simulink model "sim_pos_att3"  (R2018b)
settings: Solver=ode1  StartTime=0.0  StopTime=20  FixedStep=dt  RelTol=1e-3
values from neighbouring files (symbols this model uses):
  pitch = pitch - vel_forward_min_pitch    [forward_throttle_pct.m]
undefined symbols (not defined in the file or in its folder): GRAVITY_MSS, gyro_x, gyro_y, gyro_z, HD, Kd, Ku, Ld, Ldx, Ldy, Lu, Lux, Luy, m, p_angle_pitch, p_angle_yaw, pwm_max, pwm_min, Qd, Qu, roll, throttle_hover, yaw
libraries: shared6dof x1
(part 1 of 2)
settings Model: PauseTimes=0.5  Creator=a4327  LastModifiedBy=a4327
settings OptimizationCC: DefaultParameterBehavior=Inlined  UseDivisionForNetSlopeComputation=on  UseFloatMulNetSlope=on  InlineInvariantSignals=on  PassReuseOutputArgsAs=Individual arguments  ZeroExternalMemoryAtStartup=off  ZeroInternalMemoryAtStartup=off  NoFixptDivByZeroProtection=on  EfficientFloat2IntCast=on  LifeSpan=1  OptimizeBlockOrder=speed  DifferentSizesBufferReuse=on
settings DebuggingCC: ParameterTunabilityLossMsg=error
settings HardwareCC: ProdBitPerPointer=32  ProdBitPerSizeT=32  ProdBitPerPtrDiffT=32  ProdLargestAtomicFloat=None  ProdWordSize=32  ProdLongLongMode=on  ProdHWDeviceType=Custom Processor->Custom Processor
settings SFSimCC: MATLABDynamicMemAlloc=off
settings RTWCC: SystemTargetFile=ert.tlc  TemplateMakefile=ert_default_tmf  GenerateReport=on  IncludeHyperlinkInReport=on  LaunchReport=on  GenerateTraceInfo=on  GenerateTraceReport=on  GenerateTraceReportSl=on  GenerateTraceReportSf=on  GenerateTraceReportEml=on  GenerateCodeMetricsReport=on
settings CodeAppCC: ForceParamTrailComments=on  IgnoreCustomStorageClasses=off  OperatorAnnotations=on  SimulinkDataObjDesc=on  SFDataObjDesc=on  CustomSymbolStrGlobalVar=rt$N$M  CustomSymbolStrType=$N$M  CustomSymbolStrFcn=$N$M$F  CustomSymbolStrMacro=$N$M  InsertBlockDesc=on
settings ERTTargetCC: TargetLangStandard=C99 (ISO)  GenerateSampleERTMain=on  IncludeMdlTerminateFcn=off  CombineSignalStateStructs=on  SupportAbsoluteTime=off  MultiInstanceERTCode=on  CodeInterfacePackaging=Reusable function  SupportComplex=off  SupportNonInlinedSFcns=on  InlinedParameterPlacement=NonHierarchical  ERTCustomFileTemplate=example_file_process.tlc  ERTFilePackagingFormat=CompactWithDataFile

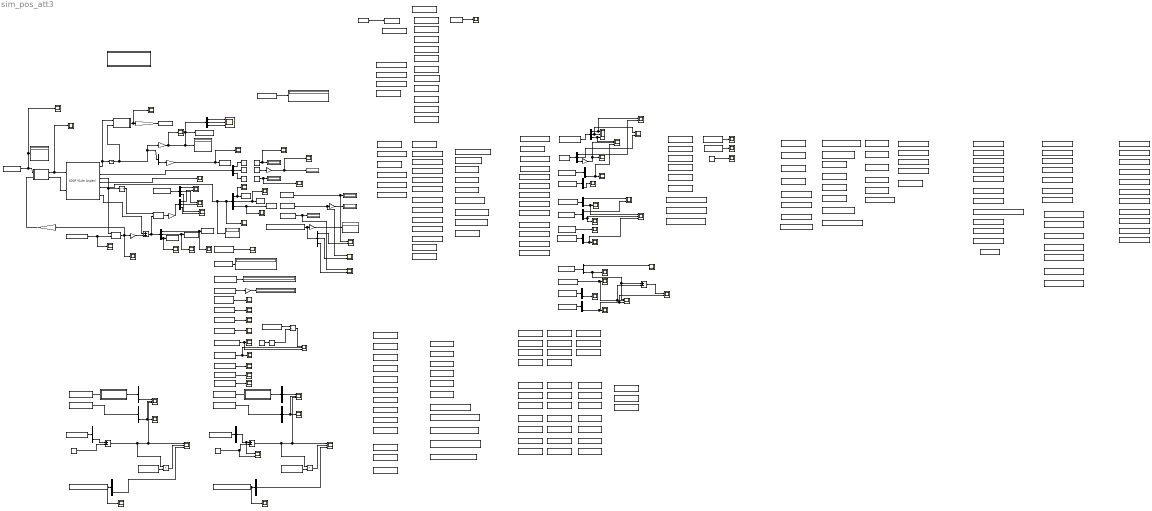
== system sim_pos_att3 ==
  6DOF (Euler Angles) : shared6dof/6DOF (Euler Angles)  units=Metric (MKS)  mtype=Fixed  rep=Euler Angles  xme_0=[0 0 0]  Vm_0=[0 0 0]  eul_0=[roll pitch yaw]  pm_0=[gyro_x gyro_y gyro_z]  mass_0=m  mass_e=0.5  mass_f=2.0  inertia=J  inertia_e=eye(3)  inertia_f=2*eye(3)  k_quat=1.0  vre_flag=on  abi_flag=off  aMode=0  xme_statename=''  Vm_statename=''  eul_statename=''  quat_statename=''  pm_statename=''  mass_statename=''
      settings: SourceProductBaseCode=AE
  AC_ATTITUDE_ACCEL_RP_CONTROLLER_MAX_RADSS : DataStoreMemory  DataStoreName=AC_ATTITUDE_ACCEL_RP_CONTROLLER_MAX_RADSS  ReadBeforeWriteMsg=warning  WriteAfterWriteMsg=warning  WriteAfterReadMsg=warning  InitialValue=AC_ATTITUDE_ACCEL_RP_CONTROLLER_MAX_RADSS  VectorParams1D=off  ShowAdditionalParam=off  OutDataTypeStr=double
  AC_ATTITUDE_ACCEL_RP_CONTROLLER_MIN_RADSS : DataStoreMemory  DataStoreName=AC_ATTITUDE_ACCEL_RP_CONTROLLER_MIN_RADSS  ReadBeforeWriteMsg=warning  WriteAfterWriteMsg=warning  WriteAfterReadMsg=warning  InitialValue=AC_ATTITUDE_ACCEL_RP_CONTROLLER_MIN_RADSS  VectorParams1D=off  ShowAdditionalParam=off  OutDataTypeStr=double
  AC_ATTITUDE_ACCEL_Y_CONTROLLER_MAX_RADSS : DataStoreMemory  DataStoreName=AC_ATTITUDE_ACCEL_Y_CONTROLLER_MAX_RADSS  ReadBeforeWriteMsg=warning  WriteAfterWriteMsg=warning  WriteAfterReadMsg=warning  InitialValue=AC_ATTITUDE_ACCEL_Y_CONTROLLER_MAX_RADSS  ShowAdditionalParam=off  OutDataTypeStr=double
  AC_ATTITUDE_ACCEL_Y_CONTROLLER_MIN_RADSS : DataStoreMemory  DataStoreName=AC_ATTITUDE_ACCEL_Y_CONTROLLER_MIN_RADSS  ReadBeforeWriteMsg=warning  WriteAfterWriteMsg=warning  WriteAfterReadMsg=warning  InitialValue=AC_ATTITUDE_ACCEL_Y_CONTROLLER_MIN_RADSS  VectorParams1D=off  ShowAdditionalParam=off  OutDataTypeStr=double
  AC_ATTITUDE_CONTROL_ANGLE_LIMIT_THROTTLE_MAX : DataStoreMemory  DataStoreName=AC_ATTITUDE_CONTROL_ANGLE_LIMIT_THROTTLE_MAX  ReadBeforeWriteMsg=warning  WriteAfterWriteMsg=warning  WriteAfterReadMsg=warning  InitialValue=AC_ATTITUDE_CONTROL_ANGLE_LIMIT_THROTTLE_MAX  VectorParams1D=off  ShowAdditionalParam=off  OutDataTypeStr=double
  AC_ATTITUDE_CONTROL_MAX : DataStoreMemory  DataStoreName=AC_ATTITUDE_CONTROL_MAX  ReadBeforeWriteMsg=warning  WriteAfterWriteMsg=warning  WriteAfterReadMsg=warning  InitialValue=AC_ATTITUDE_CONTROL_MAX  VectorParams1D=off  ShowAdditionalParam=off  OutDataTypeStr=double
  AC_ATTITUDE_THRUST_ERROR_ANGLE : DataStoreMemory  DataStoreName=AC_ATTITUDE_THRUST_ERROR_ANGLE  ReadBeforeWriteMsg=warning  WriteAfterWriteMsg=warning  WriteAfterReadMsg=warning  InitialValue=AC_ATTITUDE_THRUST_ERROR_ANGLE  ShowAdditionalParam=off  OutDataTypeStr=double
  AP_MOTORS_MATRIX_YAW_FACTOR_CCW : DataStoreMemory  DataStoreName=AP_MOTORS_MATRIX_YAW_FACTOR_CCW  ReadBeforeWriteMsg=warning  WriteAfterWriteMsg=warning  WriteAfterReadMsg=warning  InitialValue=AP_MOTORS_MATRIX_YAW_FACTOR_CCW  VectorParams1D=off  ShowAdditionalParam=off  OutDataTypeStr=double
  AP_MOTORS_MATRIX_YAW_FACTOR_CW : DataStoreMemory  DataStoreName=AP_MOTORS_MATRIX_YAW_FACTOR_CW  ReadBeforeWriteMsg=warning  WriteAfterWriteMsg=warning  WriteAfterReadMsg=warning  InitialValue=AP_MOTORS_MATRIX_YAW_FACTOR_CW  VectorParams1D=off  ShowAdditionalParam=off  OutDataTypeStr=double
  ATC_RAT_PIT_D : DataStoreMemory  DataStoreName=ATC_RAT_PIT_D  ReadBeforeWriteMsg=warning  WriteAfterWriteMsg=warning  WriteAfterReadMsg=warning  InitialValue=ATC_RAT_PIT_D  VectorParams1D=off  ShowAdditionalParam=off  OutDataTypeStr=double
  ATC_RAT_PIT_FF : DataStoreMemory  DataStoreName=ATC_RAT_PIT_FF  ReadBeforeWriteMsg=warning  WriteAfterWriteMsg=warning  WriteAfterReadMsg=warning  InitialValue=ATC_RAT_PIT_FF  VectorParams1D=off  ShowAdditionalParam=off  OutDataTypeStr=double
  ATC_RAT_PIT_FILT : DataStoreMemory  DataStoreName=ATC_RAT_PIT_FILT  ReadBeforeWriteMsg=warning  WriteAfterWriteMsg=warning  WriteAfterReadMsg=warning  InitialValue=ATC_RAT_PIT_FILT  VectorParams1D=off  ShowAdditionalParam=off  OutDataTypeStr=double
  ATC_RAT_PIT_I : DataStoreMemory  DataStoreName=ATC_RAT_PIT_I  ReadBeforeWriteMsg=warning  WriteAfterWriteMsg=warning  WriteAfterReadMsg=warning  InitialValue=ATC_RAT_PIT_I  VectorParams1D=off  ShowAdditionalParam=off  OutDataTypeStr=double
  ATC_RAT_PIT_IMAX : DataStoreMemory  DataStoreName=ATC_RAT_PIT_IMAX  ReadBeforeWriteMsg=warning  WriteAfterWriteMsg=warning  WriteAfterReadMsg=warning  InitialValue=ATC_RAT_PIT_IMAX  VectorParams1D=off  ShowAdditionalParam=off  OutDataTypeStr=double
  ATC_RAT_PIT_P : DataStoreMemory  DataStoreName=ATC_RAT_PIT_P  ReadBeforeWriteMsg=warning  WriteAfterWriteMsg=warning  WriteAfterReadMsg=warning  InitialValue=ATC_RAT_PIT_P  VectorParams1D=off  ShowAdditionalParam=off  OutDataTypeStr=double
  ATC_RAT_RLL_D : DataStoreMemory  DataStoreName=ATC_RAT_RLL_D  ReadBeforeWriteMsg=warning  WriteAfterWriteMsg=warning  WriteAfterReadMsg=warning  InitialValue=ATC_RAT_RLL_D  VectorParams1D=off  ShowAdditionalParam=off  OutDataTypeStr=double
  ATC_RAT_RLL_FF : DataStoreMemory  DataStoreName=ATC_RAT_RLL_FF  ReadBeforeWriteMsg=warning  WriteAfterWriteMsg=warning  WriteAfterReadMsg=warning  InitialValue=ATC_RAT_RLL_FF  VectorParams1D=off  ShowAdditionalParam=off  OutDataTypeStr=double
  ATC_RAT_RLL_FILT : DataStoreMemory  DataStoreName=ATC_RAT_RLL_FILT  ReadBeforeWriteMsg=warning  WriteAfterWriteMsg=warning  WriteAfterReadMsg=warning  InitialValue=ATC_RAT_RLL_FILT  VectorParams1D=off  ShowAdditionalParam=off  OutDataTypeStr=double
  ATC_RAT_RLL_I : DataStoreMemory  DataStoreName=ATC_RAT_RLL_I  ReadBeforeWriteMsg=warning  WriteAfterWriteMsg=warning  WriteAfterReadMsg=warning  InitialValue=ATC_RAT_RLL_I  VectorParams1D=off  ShowAdditionalParam=off  OutDataTypeStr=double
  ATC_RAT_RLL_IMAX : DataStoreMemory  DataStoreName=ATC_RAT_RLL_IMAX  ReadBeforeWriteMsg=warning  WriteAfterWriteMsg=warning  WriteAfterReadMsg=warning  InitialValue=ATC_RAT_RLL_IMAX  VectorParams1D=off  ShowAdditionalParam=off  OutDataTypeStr=double
  ATC_RAT_RLL_P : DataStoreMemory  DataStoreName=ATC_RAT_RLL_P  ReadBeforeWriteMsg=warning  WriteAfterWriteMsg=warning  WriteAfterReadMsg=warning  InitialValue=ATC_RAT_RLL_P  VectorParams1D=off  ShowAdditionalParam=off  OutDataTypeStr=double
  ATC_RAT_YAW_D : DataStoreMemory  DataStoreName=ATC_RAT_YAW_D  ReadBeforeWriteMsg=warning  WriteAfterWriteMsg=warning  WriteAfterReadMsg=warning  InitialValue=ATC_RAT_YAW_D  VectorParams1D=off  ShowAdditionalParam=off  OutDataTypeStr=double
  ATC_RAT_YAW_FF : DataStoreMemory  DataStoreName=ATC_RAT_YAW_FF  ReadBeforeWriteMsg=warning  WriteAfterWriteMsg=warning  WriteAfterReadMsg=warning  InitialValue=ATC_RAT_YAW_FF  VectorParams1D=off  ShowAdditionalParam=off  OutDataTypeStr=double
  ATC_RAT_YAW_FILT : DataStoreMemory  DataStoreName=ATC_RAT_YAW_FILT  ReadBeforeWriteMsg=warning  WriteAfterWriteMsg=warning  WriteAfterReadMsg=warning  InitialValue=ATC_RAT_YAW_FILT  VectorParams1D=off  ShowAdditionalParam=off  OutDataTypeStr=double
  ATC_RAT_YAW_I : DataStoreMemory  DataStoreName=ATC_RAT_YAW_I  ReadBeforeWriteMsg=warning  WriteAfterWriteMsg=warning  WriteAfterReadMsg=warning  InitialValue=ATC_RAT_YAW_I  VectorParams1D=off  ShowAdditionalParam=off  OutDataTypeStr=double
  ATC_RAT_YAW_IMAX : DataStoreMemory  DataStoreName=ATC_RAT_YAW_IMAX  ReadBeforeWriteMsg=warning  WriteAfterWriteMsg=warning  WriteAfterReadMsg=warning  InitialValue=ATC_RAT_YAW_IMAX  VectorParams1D=off  ShowAdditionalParam=off  OutDataTypeStr=double
  ATC_RAT_YAW_P : DataStoreMemory  DataStoreName=ATC_RAT_YAW_P  ReadBeforeWriteMsg=warning  WriteAfterWriteMsg=warning  WriteAfterReadMsg=warning  InitialValue=ATC_RAT_YAW_P  VectorParams1D=off  ShowAdditionalParam=off  OutDataTypeStr=double
  Add : Sum  Inputs=+-
  Add1 : Sum  Inputs=+-
  Add2 : Sum  Inputs=+-
  Add3 : Sum
  Constant : Constant  Value=p_angle_pitch
  Constant1 : Constant  Value=p_angle_yaw
  Constant2 : Constant  Value=throttle_hover
  Constant3 : Constant  Value=0.4816
  Cos : Trigonometry  Operator=cos
  Data Store Read : DataStoreRead  DataStoreName=pwm_out
  Data Store Read1 : DataStoreRead  DataStoreName=pitch
  Data Store Read10 : DataStoreRead  DataStoreName=gyro_y
  Data Store Read11 : DataStoreRead  DataStoreName=gyro_z
  Data Store Read{9,12,26,31} (4 alike) : DataStoreRead  DataStoreName=rate_target_ang_vel
  Data Store Read13 : DataStoreRead  DataStoreName=pitch_in
  Data Store Read14 : DataStoreRead  DataStoreName=roll_in
  Data Store Read15 : DataStoreRead  DataStoreName=yaw_in
  Data Store Read16 : DataStoreRead  DataStoreName=throttle_filter
  Data Store Read17 : DataStoreRead  DataStoreName=thrust_rpyt_out
  Data Store Read{7,18,25,30} (4 alike) : DataStoreRead  DataStoreName=attitude_target_euler_angle
  Data Store Read19 : DataStoreRead  DataStoreName=throttle_in
  Data Store Read2 : DataStoreRead  DataStoreName=roll
  Data Store Read20 : DataStoreRead  DataStoreName=attitude_target_euler_rate
  Data Store Read21 : DataStoreRead  DataStoreName=attitude_target_ang_vel
  Data Store Read22 : DataStoreRead  DataStoreName=attitude_ang_error
  Data Store Read23 : DataStoreRead  DataStoreName=attitude_error_vector
  Data Store Read24 : DataStoreRead  DataStoreName=pitch
  Data Store Read27 : DataStoreRead  DataStoreName=attitude_ang_error
  Data Store Read28 : DataStoreRead  DataStoreName=attitude_error_vector
  Data Store Read29 : DataStoreRead  DataStoreName=yaw
  Data Store Read3 : DataStoreRead  DataStoreName=yaw
  Data Store Read32 : DataStoreRead  DataStoreName=leash_up_z
  Data Store Read33 : DataStoreRead  DataStoreName=leash_down_z
  Data Store Read34 : DataStoreRead  DataStoreName=pos_target
  Data Store Read35 : DataStoreRead  DataStoreName=accel_target
  Data Store Read36 : DataStoreRead  DataStoreName=pos_error
  Data Store Read37 : DataStoreRead  DataStoreName=vel_target
  Data Store Read38 : DataStoreRead  DataStoreName=curr_vel
  Data Store Read39 : DataStoreRead  DataStoreName=vel_desired
  Data Store Read4 : DataStoreRead  DataStoreName=rot_body_to_ned
  Data Store Read40 : DataStoreRead  DataStoreName=vel_last
  Data Store Read41 : DataStoreRead  DataStoreName=vel_error
  Data Store Read42 : DataStoreRead  DataStoreName=accel_target
  Data Store Read43 : DataStoreRead  DataStoreName=z_accel_meas
  Data Store Read44 : DataStoreRead  DataStoreName=accel_desired
  Data Store Read45 : DataStoreRead  DataStoreName=accel_error
  Data Store Read46 : DataStoreRead  DataStoreName=leash
  Data Store Read47 : DataStoreRead  DataStoreName=angle_boost
  Data Store Read48 : DataStoreRead  DataStoreName=pitch
  Data Store Read49 : DataStoreRead  DataStoreName=throttle_in
  Data Store Read5 : DataStoreRead  DataStoreName=rot_body_to_ned
  Data Store Read50 : DataStoreRead  DataStoreName=curr_pos
  Data Store Read6 : DataStoreRead  DataStoreName=attitude_target_quat
  Data Store Read8 : DataStoreRead  DataStoreName=gyro_x
  Data Store Write : DataStoreWrite  DataStoreName=throttle_in
  Data Store Write1 : DataStoreWrite  DataStoreName=roll
  Data Store Write10 : DataStoreWrite  DataStoreName=curr_pos
  Data Store Write11 : DataStoreWrite  DataStoreName=accel_y
  Data Store Write12 : DataStoreWrite  DataStoreName=accel_x
  Data Store Write2 : DataStoreWrite  DataStoreName=yaw
  Data Store Write3 : DataStoreWrite  DataStoreName=pitch
  Data Store Write4 : DataStoreWrite  DataStoreName=gyro_x
  Data Store Write5 : DataStoreWrite  DataStoreName=gyro_y
  Data Store Write6 : DataStoreWrite  DataStoreName=gyro_z
  Data Store Write7 : DataStoreWrite  DataStoreName=curr_alt
  Data Store Write8 : DataStoreWrite  DataStoreName=accel_z
  Data Store Write9 : DataStoreWrite  DataStoreName=curr_vel
  Demux{,1..25} (26 alike) : Demux  Outputs=3
  Display{1..2,4..5,7,10..18} (14 alike) : Display
      Display7 settings: Format=bank
  Divide : Product  Inputs=*/
  GRAVITY_MSS : DataStoreMemory  DataStoreName=GRAVITY_MSS  ReadBeforeWriteMsg=warning  WriteAfterWriteMsg=warning  WriteAfterReadMsg=warning  InitialValue=GRAVITY_MSS  VectorParams1D=off  ShowAdditionalParam=off  OutDataTypeStr=double
  Gain{,1..3} (4 alike) : Gain  Gain=HD
  Gain4 : Gain  Gain=-100
  Gain5 : Gain  Gain=[100 100 -100]
  Gain6 : Gain  Gain=-1
  Gain7 : Gain  Gain=100
  Gain8 : Gain  Gain=-1
  Gain9 : Gain  Gain=100
  Gravity in Earth Axes : Gain  Gain=m  SaturateOnIntegerOverflow=on  OutDataTypeStr=Inherit: Same as input  ParamDataTypeStr=Inherit: Same as input
  Inertial to Body : Product  Multiplication=Matrix(*)  SaturateOnIntegerOverflow=on  InputSameDT=on  OutDataTypeStr=Inherit: Same as first input
  Inertial to NED : Product  Multiplication=Matrix(*)  SaturateOnIntegerOverflow=on  InputSameDT=on  OutDataTypeStr=Inherit: Same as first input
  Kx : DataStoreMemory  DataStoreName=Kx  ReadBeforeWriteMsg=warning  WriteAfterWriteMsg=warning  WriteAfterReadMsg=warning  InitialValue=Kx  VectorParams1D=off  ShowAdditionalParam=off  OutDataTypeStr=double
  MATLAB Function : MATLAB Function  TreatAsAtomicUnit=on
  MATLAB Function1 : MATLAB Function  TreatAsAtomicUnit=on
  MATLAB Function2 : MATLAB Function  TreatAsAtomicUnit=on
  POSCONTROL_ACCELERATION_MIN : DataStoreMemory  DataStoreName=POSCONTROL_ACCELERATION_MIN  ReadBeforeWriteMsg=warning  WriteAfterWriteMsg=warning  WriteAfterReadMsg=warning  InitialValue=POSCONTROL_ACCELERATION_MIN  ShowAdditionalParam=off  OutDataTypeStr=double
  POSCONTROL_ACCEL_FILTER_HZ : DataStoreMemory  DataStoreName=POSCONTROL_ACCEL_FILTER_HZ  ReadBeforeWriteMsg=warning  WriteAfterWriteMsg=warning  WriteAfterReadMsg=warning  InitialValue=POSCONTROL_ACCEL_FILTER_HZ  VectorParams1D=off  ShowAdditionalParam=off  OutDataTypeStr=double
  POSCONTROL_ACCEL_XY : DataStoreMemory  DataStoreName=POSCONTROL_ACCEL_XY  ReadBeforeWriteMsg=warning  WriteAfterWriteMsg=warning  WriteAfterReadMsg=warning  InitialValue=POSCONTROL_ACCEL_XY  VectorParams1D=off  ShowAdditionalParam=off  OutDataTypeStr=double
  POSCONTROL_ACCEL_XY_MAX : DataStoreMemory  DataStoreName=POSCONTROL_ACCEL_XY_MAX  ReadBeforeWriteMsg=warning  WriteAfterWriteMsg=warning  WriteAfterReadMsg=warning  InitialValue=POSCONTROL_ACCEL_XY_MAX  VectorParams1D=off  ShowAdditionalParam=off  OutDataTypeStr=double
  POSCONTROL_ACCEL_Z : DataStoreMemory  DataStoreName=POSCONTROL_ACCEL_Z  ReadBeforeWriteMsg=warning  WriteAfterWriteMsg=warning  WriteAfterReadMsg=warning  InitialValue=POSCONTROL_ACCEL_Z  ShowAdditionalParam=off  OutDataTypeStr=double
  POSCONTROL_ACC_Z_D : DataStoreMemory  DataStoreName=POSCONTROL_ACC_Z_D  ReadBeforeWriteMsg=warning  WriteAfterWriteMsg=warning  WriteAfterReadMsg=warning  InitialValue=POSCONTROL_ACC_Z_D  VectorParams1D=off  ShowAdditionalParam=off  OutDataTypeStr=double
  POSCONTROL_ACC_Z_FILT_HZ : DataStoreMemory  DataStoreName=POSCONTROL_ACC_Z_FILT_HZ  ReadBeforeWriteMsg=warning  WriteAfterWriteMsg=warning  WriteAfterReadMsg=warning  InitialValue=POSCONTROL_ACC_Z_FILT_HZ  VectorParams1D=off  ShowAdditionalParam=off  OutDataTypeStr=double
  POSCONTROL_ACC_Z_I : DataStoreMemory  DataStoreName=POSCONTROL_ACC_Z_I  ReadBeforeWriteMsg=warning  WriteAfterWriteMsg=warning  WriteAfterReadMsg=warning  InitialValue=POSCONTROL_ACC_Z_I  VectorParams1D=off  ShowAdditionalParam=off  OutDataTypeStr=double
  POSCONTROL_ACC_Z_IMAX : DataStoreMemory  DataStoreName=POSCONTROL_ACC_Z_IMAX  ReadBeforeWriteMsg=warning  WriteAfterWriteMsg=warning  WriteAfterReadMsg=warning  InitialValue=POSCONTROL_ACC_Z_IMAX  VectorParams1D=off  ShowAdditionalParam=off  OutDataTypeStr=double
  POSCONTROL_ACC_Z_P : DataStoreMemory  DataStoreName=POSCONTROL_ACC_Z_P  ReadBeforeWriteMsg=warning  WriteAfterWriteMsg=warning  WriteAfterReadMsg=warning  InitialValue=POSCONTROL_ACC_Z_P  VectorParams1D=off  ShowAdditionalParam=off  OutDataTypeStr=double
  POSCONTROL_JERK_RATIO : DataStoreMemory  DataStoreName=POSCONTROL_JERK_RATIO  ReadBeforeWriteMsg=warning  WriteAfterWriteMsg=warning  WriteAfterReadMsg=warning  InitialValue=POSCONTROL_JERK_RATIO  VectorParams1D=off  ShowAdditionalParam=off  OutDataTypeStr=double
  POSCONTROL_LEASH_LENGTH_MIN : DataStoreMemory  DataStoreName=POSCONTROL_LEASH_LENGTH_MIN  ReadBeforeWriteMsg=warning  WriteAfterWriteMsg=warning  WriteAfterReadMsg=warning  InitialValue=POSCONTROL_LEASH_LENGTH_MIN  VectorParams1D=off  ShowAdditionalParam=off  OutDataTypeStr=double
  POSCONTROL_OVERSPEED_GAIN_Z : DataStoreMemory  DataStoreName=POSCONTROL_OVERSPEED_GAIN_Z  ReadBeforeWriteMsg=warning  WriteAfterWriteMsg=warning  WriteAfterReadMsg=warning  InitialValue=POSCONTROL_OVERSPEED_GAIN_Z  VectorParams1D=off  ShowAdditionalParam=off  OutDataTypeStr=double
  POSCONTROL_POS_XY_P : DataStoreMemory  DataStoreName=POSCONTROL_POS_XY_P  ReadBeforeWriteMsg=warning  WriteAfterWriteMsg=warning  WriteAfterReadMsg=warning  InitialValue=POSCONTROL_POS_XY_P  VectorParams1D=off  ShowAdditionalParam=off  OutDataTypeStr=double
  POSCONTROL_POS_Z_P : DataStoreMemory  DataStoreName=POSCONTROL_POS_Z_P  ReadBeforeWriteMsg=warning  WriteAfterWriteMsg=warning  WriteAfterReadMsg=warning  InitialValue=POSCONTROL_POS_Z_P  VectorParams1D=off  ShowAdditionalParam=off  OutDataTypeStr=double
  POSCONTROL_SPEED : DataStoreMemory  DataStoreName=POSCONTROL_SPEED  ReadBeforeWriteMsg=warning  WriteAfterWriteMsg=warning  WriteAfterReadMsg=warning  InitialValue=POSCONTROL_SPEED  ShowAdditionalParam=off  OutDataTypeStr=double
  POSCONTROL_SPEED_DOWN : DataStoreMemory  DataStoreName=POSCONTROL_SPEED_DOWN  ReadBeforeWriteMsg=warning  WriteAfterWriteMsg=warning  WriteAfterReadMsg=warning  InitialValue=POSCONTROL_SPEED_DOWN  ShowAdditionalParam=off  OutDataTypeStr=double
  POSCONTROL_SPEED_UP : DataStoreMemory  DataStoreName=POSCONTROL_SPEED_UP  ReadBeforeWriteMsg=warning  WriteAfterWriteMsg=warning  WriteAfterReadMsg=warning  InitialValue=POSCONTROL_SPEED_UP  ShowAdditionalParam=off  OutDataTypeStr=double
  POSCONTROL_STOPPING_DIST_DOWN_MAX : DataStoreMemory  DataStoreName=POSCONTROL_STOPPING_DIST_DOWN_MAX  ReadBeforeWriteMsg=warning  WriteAfterWriteMsg=warning  WriteAfterReadMsg=warning  InitialValue=POSCONTROL_STOPPING_DIST_DOWN_MAX  VectorParams1D=off  ShowAdditionalParam=off  OutDataTypeStr=double
  POSCONTROL_STOPPING_DIST_UP_MAX : DataStoreMemory  DataStoreName=POSCONTROL_STOPPING_DIST_UP_MAX  ReadBeforeWriteMsg=warning  WriteAfterWriteMsg=warning  WriteAfterReadMsg=warning  InitialValue=POSCONTROL_STOPPING_DIST_UP_MAX  VectorParams1D=off  ShowAdditionalParam=off  OutDataTypeStr=double
  POSCONTROL_THROTTLE_CUTOFF_FREQ : DataStoreMemory  DataStoreName=POSCONTROL_THROTTLE_CUTOFF_FREQ  ReadBeforeWriteMsg=warning  WriteAfterWriteMsg=warning  WriteAfterReadMsg=warning  InitialValue=POSCONTROL_THROTTLE_CUTOFF_FREQ  VectorParams1D=off  ShowAdditionalParam=off  OutDataTypeStr=double
  POSCONTROL_VEL_ERROR_CUTOFF_FREQ : DataStoreMemory  DataStoreName=POSCONTROL_VEL_ERROR_CUTOFF_FREQ  ReadBeforeWriteMsg=warning  WriteAfterWriteMsg=warning  WriteAfterReadMsg=warning  InitialValue=POSCONTROL_VEL_ERROR_CUTOFF_FREQ  VectorParams1D=off  ShowAdditionalParam=off  OutDataTypeStr=double
  POSCONTROL_VEL_XY_D : DataStoreMemory  DataStoreName=POSCONTROL_VEL_XY_D  ReadBeforeWriteMsg=warning  WriteAfterWriteMsg=warning  WriteAfterReadMsg=warning  InitialValue=POSCONTROL_VEL_XY_D  VectorParams1D=off  ShowAdditionalParam=off  OutDataTypeStr=double
  POSCONTROL_VEL_XY_FILT_D_HZ : DataStoreMemory  DataStoreName=POSCONTROL_VEL_XY_FILT_D_HZ  ReadBeforeWriteMsg=warning  WriteAfterWriteMsg=warning  WriteAfterReadMsg=warning  InitialValue=POSCONTROL_VEL_XY_FILT_D_HZ  VectorParams1D=off  ShowAdditionalParam=off  OutDataTypeStr=double
  POSCONTROL_VEL_XY_FILT_HZ : DataStoreMemory  DataStoreName=POSCONTROL_VEL_XY_FILT_HZ  ReadBeforeWriteMsg=warning  WriteAfterWriteMsg=warning  WriteAfterReadMsg=warning  InitialValue=POSCONTROL_VEL_XY_FILT_HZ  VectorParams1D=off  ShowAdditionalParam=off  OutDataTypeStr=double
  POSCONTROL_VEL_XY_I : DataStoreMemory  DataStoreName=POSCONTROL_VEL_XY_I  ReadBeforeWriteMsg=warning  WriteAfterWriteMsg=warning  WriteAfterReadMsg=warning  InitialValue=POSCONTROL_VEL_XY_I  VectorParams1D=off  ShowAdditionalParam=off  OutDataTypeStr=double
  POSCONTROL_VEL_XY_IMAX : DataStoreMemory  DataStoreName=POSCONTROL_VEL_XY_IMAX  ReadBeforeWriteMsg=warning  WriteAfterWriteMsg=warning  WriteAfterReadMsg=warning  InitialValue=POSCONTROL_VEL_XY_IMAX  VectorParams1D=off  ShowAdditionalParam=off  OutDataTypeStr=double
  POSCONTROL_VEL_XY_P : DataStoreMemory  DataStoreName=POSCONTROL_VEL_XY_P  ReadBeforeWriteMsg=warning  WriteAfterWriteMsg=warning  WriteAfterReadMsg=warning  InitialValue=POSCONTROL_VEL_XY_P  VectorParams1D=off  ShowAdditionalParam=off  OutDataTypeStr=double
  POSCONTROL_VEL_Z_P : DataStoreMemory  DataStoreName=POSCONTROL_VEL_Z_P  ReadBeforeWriteMsg=warning  WriteAfterWriteMsg=warning  WriteAfterReadMsg=warning  InitialValue=POSCONTROL_VEL_Z_P  VectorParams1D=off  ShowAdditionalParam=off  OutDataTypeStr=double
  Product : Product
  Product1 : Product
  Scope{,1,3..13,15..17,19,21,23..24,27,29..32,34..37,39..46,48..50,54..55,58..59,61..62,64} (47 alike) : Scope
  Scope{2,14,22,25,47,52,57,63,65..68} (12 alike) : Scope  NumInputPorts=2
  Scope{18,20,26,28,33,38,51,53,56,60} (10 alike) : Scope  NumInputPorts=3
  Transpose : Math  Operator=transpose  SaturateOnIntegerOverflow=on
  accel_desired : DataStoreMemory  DataStoreName=accel_desired  ReadBeforeWriteMsg=warning  WriteAfterWriteMsg=warning  WriteAfterReadMsg=warning  InitialValue=accel_desired  VectorParams1D=off  ShowAdditionalParam=off  OutDataTypeStr=double
  accel_error : DataStoreMemory  DataStoreName=accel_error  ReadBeforeWriteMsg=warning  WriteAfterWriteMsg=warning  WriteAfterReadMsg=warning  InitialValue=accel_error  VectorParams1D=off  ShowAdditionalParam=off  OutDataTypeStr=double
  accel_last_z_cms : DataStoreMemory  DataStoreName=accel_last_z_cms  ReadBeforeWriteMsg=warning  WriteAfterWriteMsg=warning  WriteAfterReadMsg=warning  InitialValue=accel_last_z_cms  VectorParams1D=off  ShowAdditionalParam=off  OutDataTypeStr=double
  accel_pitch_max : DataStoreMemory  DataStoreName=accel_pitch_max  ReadBeforeWriteMsg=warning  WriteAfterWriteMsg=warning  WriteAfterReadMsg=warning  InitialValue=accel_pitch_max  VectorParams1D=off  ShowAdditionalParam=off  OutDataTypeStr=double
  accel_roll_max : DataStoreMemory  DataStoreName=accel_roll_max  ReadBeforeWriteMsg=warning  WriteAfterWriteMsg=warning  WriteAfterReadMsg=warning  InitialValue=accel_roll_max  VectorParams1D=off  ShowAdditionalParam=off  OutDataTypeStr=double
  accel_target : DataStoreMemory  DataStoreName=accel_target  ReadBeforeWriteMsg=warning  WriteAfterWriteMsg=warning  WriteAfterReadMsg=warning  InitialValue=accel_target  VectorParams1D=off  ShowAdditionalParam=off  OutDataTypeStr=double
  accel_x : DataStoreMemory  DataStoreName=accel_x  ReadBeforeWriteMsg=warning  WriteAfterWriteMsg=warning  WriteAfterReadMsg=warning  InitialValue=accel_x  ShowAdditionalParam=off  OutDataTypeStr=double
  accel_xy_angle_max : DataStoreMemory  DataStoreName=accel_xy_angle_max  ReadBeforeWriteMsg=warning  WriteAfterWriteMsg=warning  WriteAfterReadMsg=warning  InitialValue=accel_xy_angle_max  VectorParams1D=off  ShowAdditionalParam=off  OutDataTypeStr=double
  accel_xy_input : DataStoreMemory  DataStoreName=accel_xy_input  ReadBeforeWriteMsg=warning  WriteAfterWriteMsg=warning  WriteAfterReadMsg=warning  InitialValue=accel_xy_input  VectorParams1D=off  ShowAdditionalParam=off  OutDataTypeStr=double
  accel_y : DataStoreMemory  DataStoreName=accel_y  ReadBeforeWriteMsg=warning  WriteAfterWriteMsg=warning  WriteAfterReadMsg=warning  InitialValue=accel_y  ShowAdditionalParam=off  OutDataTypeStr=double
  accel_yaw_max : DataStoreMemory  DataStoreName=accel_yaw_max  ReadBeforeWriteMsg=warning  WriteAfterWriteMsg=warning  WriteAfterReadMsg=warning  InitialValue=accel_yaw_max  VectorParams1D=off  ShowAdditionalParam=off  OutDataTypeStr=double
  accel_z : DataStoreMemory  DataStoreName=accel_z  ReadBeforeWriteMsg=warning  WriteAfterWriteMsg=warning  WriteAfterReadMsg=warning  InitialValue=accel_z  ShowAdditionalParam=off  OutDataTypeStr=double
  air_density_ratio : DataStoreMemory  DataStoreName=air_density_ratio  ReadBeforeWriteMsg=warning  WriteAfterWriteMsg=warning  WriteAfterReadMsg=warning  InitialValue=air_density_ratio  VectorParams1D=off  ShowAdditionalParam=off  OutDataTypeStr=double
  althold_lean_angle_max : DataStoreMemory  DataStoreName=althold_lean_angle_max  ReadBeforeWriteMsg=warning  WriteAfterWriteMsg=warning  WriteAfterReadMsg=warning  InitialValue=althold_lean_angle_max  VectorParams1D=off  ShowAdditionalParam=off  OutDataTypeStr=double
  ang_vel_pitch_max : DataStoreMemory  DataStoreName=ang_vel_pitch_max  ReadBeforeWriteMsg=warning  WriteAfterWriteMsg=warning  WriteAfterReadMsg=warning  InitialValue=ang_vel_pitch_max  ShowAdditionalParam=off  OutDataTypeStr=double
  ang_vel_roll_max : DataStoreMemory  DataStoreName=ang_vel_roll_max  ReadBeforeWriteMsg=warning  WriteAfterWriteMsg=warning  WriteAfterReadMsg=warning  InitialValue=ang_vel_roll_max  ShowAdditionalParam=off  OutDataTypeStr=double
  ang_vel_yaw_max : DataStoreMemory  DataStoreName=ang_vel_yaw_max  ReadBeforeWriteMsg=warning  WriteAfterWriteMsg=warning  WriteAfterReadMsg=warning  InitialValue=ang_vel_yaw_max  ShowAdditionalParam=off  OutDataTypeStr=double
  angle_boost : DataStoreMemory  DataStoreName=angle_boost  ReadBeforeWriteMsg=warning  WriteAfterWriteMsg=warning  WriteAfterReadMsg=warning  InitialValue=angle_boost  VectorParams1D=off  ShowAdditionalParam=off  OutDataTypeStr=double
  angle_boost_enabled : DataStoreMemory  DataStoreName=angle_boost_enabled  ReadBeforeWriteMsg=warning  WriteAfterWriteMsg=warning  WriteAfterReadMsg=warning  InitialValue=angle_boost_enabled  VectorParams1D=off  ShowAdditionalParam=off  OutDataTypeStr=double
  angle_limit_tc : DataStoreMemory  DataStoreName=angle_limit_tc  ReadBeforeWriteMsg=warning  WriteAfterWriteMsg=warning  WriteAfterReadMsg=warning  InitialValue=angle_limit_tc  VectorParams1D=off  ShowAdditionalParam=off  OutDataTypeStr=double
  armed : DataStoreMemory  DataStoreName=armed  ReadBeforeWriteMsg=warning  WriteAfterWriteMsg=warning  WriteAfterReadMsg=warning  InitialValue=armed  VectorParams1D=off  ShowAdditionalParam=off  OutDataTypeStr=double
  attitude_ang_error : DataStoreMemory  DataStoreName=attitude_ang_error  ReadBeforeWriteMsg=warning  WriteAfterWriteMsg=warning  WriteAfterReadMsg=warning  InitialValue=attitude_ang_error  VectorParams1D=off  ShowAdditionalParam=off  OutDataTypeStr=double
  attitude_error_vector : DataStoreMemory  DataStoreName=attitude_error_vector  ReadBeforeWriteMsg=warning  WriteAfterWriteMsg=warning  WriteAfterReadMsg=warning  InitialValue=attitude_error_vector  VectorParams1D=off  ShowAdditionalParam=off  OutDataTypeStr=double
  attitude_target_ang_vel : DataStoreMemory  DataStoreName=attitude_target_ang_vel  ReadBeforeWriteMsg=warning  WriteAfterWriteMsg=warning  WriteAfterReadMsg=warning  InitialValue=attitude_target_ang_vel  VectorParams1D=off  ShowAdditionalParam=off  OutDataTypeStr=double
  attitude_target_euler_angle : DataStoreMemory  DataStoreName=attitude_target_euler_angle  ReadBeforeWriteMsg=warning  WriteAfterWriteMsg=warning  WriteAfterReadMsg=warning  InitialValue=attitude_target_euler_angle  VectorParams1D=off  ShowAdditionalParam=off  OutDataTypeStr=double
  attitude_target_euler_rate : DataStoreMemory  DataStoreName=attitude_target_euler_rate  ReadBeforeWriteMsg=warning  WriteAfterWriteMsg=warning  WriteAfterReadMsg=warning  InitialValue=attitude_target_euler_rate  VectorParams1D=off  ShowAdditionalParam=off  OutDataTypeStr=double
  attitude_target_quat : DataStoreMemory  DataStoreName=attitude_target_quat  ReadBeforeWriteMsg=warning  WriteAfterWriteMsg=warning  WriteAfterReadMsg=warning  InitialValue=attitude_target_quat  VectorParams1D=off  ShowAdditionalParam=off  OutDataTypeStr=double
  climb_rate_cms : DataStoreMemory  DataStoreName=climb_rate_cms  ReadBeforeWriteMsg=warning  WriteAfterWriteMsg=warning  WriteAfterReadMsg=warning  InitialValue=climb_rate_cms  VectorParams1D=off  ShowAdditionalParam=off  OutDataTypeStr=double
  curr_alt : DataStoreMemory  DataStoreName=curr_alt  ReadBeforeWriteMsg=warning  WriteAfterWriteMsg=warning  WriteAfterReadMsg=warning  InitialValue=curr_alt  VectorParams1D=off  ShowAdditionalParam=off  OutDataTypeStr=double
  curr_pos : DataStoreMemory  DataStoreName=curr_pos  ReadBeforeWriteMsg=warning  WriteAfterWriteMsg=warning  WriteAfterReadMsg=warning  InitialValue=curr_pos  ShowAdditionalParam=off  OutDataTypeStr=double
  curr_vel : DataStoreMemory  DataStoreName=curr_vel  ReadBeforeWriteMsg=warning  WriteAfterWriteMsg=warning  WriteAfterReadMsg=warning  InitialValue=curr_vel  VectorParams1D=off  ShowAdditionalParam=off  OutDataTypeStr=double
  curr_vel_limt : MATLAB Function  TreatAsAtomicUnit=on
  current_tilt : DataStoreMemory  DataStoreName=current_tilt  ReadBeforeWriteMsg=warning  WriteAfterWriteMsg=warning  WriteAfterReadMsg=warning  InitialValue=current_tilt  VectorParams1D=off  ShowAdditionalParam=off  OutDataTypeStr=double
  dt : DataStoreMemory  DataStoreName=dt  ReadBeforeWriteMsg=warning  WriteAfterWriteMsg=warning  WriteAfterReadMsg=warning  InitialValue=dt  ShowAdditionalParam=off  OutDataTypeStr=double
  freeze_ff_z : DataStoreMemory  DataStoreName=freeze_ff_z  ReadBeforeWriteMsg=warning  WriteAfterWriteMsg=warning  WriteAfterReadMsg=warning  InitialValue=freeze_ff_z  VectorParams1D=off  ShowAdditionalParam=off  OutDataTypeStr=double
  gn : Constant  Value=[0;0;GRAVITY_MSS]
  gyro_x : DataStoreMemory  DataStoreName=gyro_x  ReadBeforeWriteMsg=warning  WriteAfterWriteMsg=warning  WriteAfterReadMsg=warning  InitialValue=gyro_x  ShowAdditionalParam=off  OutDataTypeStr=double
  gyro_y : DataStoreMemory  DataStoreName=gyro_y  ReadBeforeWriteMsg=warning  WriteAfterWriteMsg=warning  WriteAfterReadMsg=warning  InitialValue=gyro_y  ShowAdditionalParam=off  OutDataTypeStr=double
  gyro_z : DataStoreMemory  DataStoreName=gyro_z  ReadBeforeWriteMsg=warning  WriteAfterWriteMsg=warning  WriteAfterReadMsg=warning  InitialValue=gyro_z  ShowAdditionalParam=off  OutDataTypeStr=double
  inint : DataStoreMemory  DataStoreName=inint  ReadBeforeWriteMsg=warning  WriteAfterWriteMsg=warning  WriteAfterReadMsg=warning  InitialValue=inint  VectorParams1D=off  ShowAdditionalParam=off  OutDataTypeStr=double
  input_euler_angle_roll_pitch_euler_rate_yaw : MATLAB Function  TreatAsAtomicUnit=on
  input_tc : DataStoreMemory  DataStoreName=input_tc  ReadBeforeWriteMsg=warning  WriteAfterWriteMsg=warning  WriteAfterReadMsg=warning  InitialValue=input_tc  VectorParams1D=off  ShowAdditionalParam=off  OutDataTypeStr=double
  is_active_xy : DataStoreMemory  DataStoreName=is_active_xy  ReadBeforeWriteMsg=warning  WriteAfterWriteMsg=warning  WriteAfterReadMsg=warning  InitialValue=is_active_xy  VectorParams1D=off  ShowAdditionalParam=off  OutDataTypeStr=double
  is_active_z : DataStoreMemory  DataStoreName=is_active_z  ReadBeforeWriteMsg=warning  WriteAfterWriteMsg=warning  WriteAfterReadMsg=warning  InitialValue=is_active_z  VectorParams1D=off  ShowAdditionalParam=off  OutDataTypeStr=double
  leash : DataStoreMemory  DataStoreName=leash  ReadBeforeWriteMsg=warning  WriteAfterWriteMsg=warning  WriteAfterReadMsg=warning  InitialValue=POSCONTROL_LEASH_LENGTH_MIN  ShowAdditionalParam=off  OutDataTypeStr=double
  leash_down_z : DataStoreMemory  DataStoreName=leash_down_z  ReadBeforeWriteMsg=warning  WriteAfterWriteMsg=warning  WriteAfterReadMsg=warning  InitialValue=POSCONTROL_LEASH_LENGTH_MIN  ShowAdditionalParam=off  OutDataTypeStr=double
  leash_up_z : DataStoreMemory  DataStoreName=leash_up_z  ReadBeforeWriteMsg=warning  WriteAfterWriteMsg=warning  WriteAfterReadMsg=warning  InitialValue=POSCONTROL_LEASH_LENGTH_MIN  ShowAdditionalParam=off  OutDataTypeStr=double
  limit_accel_xy : DataStoreMemory  DataStoreName=limit_accel_xy  ReadBeforeWriteMsg=warning  WriteAfterWriteMsg=warning  WriteAfterReadMsg=warning  InitialValue=limit_accel_xy  VectorParams1D=off  ShowAdditionalParam=off  OutDataTypeStr=double
  limit_pos_down : DataStoreMemory  DataStoreName=limit_pos_down  ReadBeforeWriteMsg=warning  WriteAfterWriteMsg=warning  WriteAfterReadMsg=warning  InitialValue=limit_pos_down  VectorParams1D=off  ShowAdditionalParam=off  OutDataTypeStr=double
  limit_pos_up : DataStoreMemory  DataStoreName=limit_pos_up  ReadBeforeWriteMsg=warning  WriteAfterWriteMsg=warning  WriteAfterReadMsg=warning  InitialValue=limit_pos_up  VectorParams1D=off  ShowAdditionalParam=off  OutDataTypeStr=double
  limit_roll_pitch : DataStoreMemory  DataStoreName=limit_roll_pitch  ReadBeforeWriteMsg=warning  WriteAfterWriteMsg=warning  WriteAfterReadMsg=warning  InitialValue=limit_roll_pitch  VectorParams1D=off  ShowAdditionalParam=off  OutDataTypeStr=double
  limit_vel_down : DataStoreMemory  DataStoreName=limit_vel_down  ReadBeforeWriteMsg=warning  WriteAfterWriteMsg=warning  WriteAfterReadMsg=warning  InitialValue=limit_vel_down  VectorParams1D=off  ShowAdditionalParam=off  OutDataTypeStr=double
  limit_vel_up : DataStoreMemory  DataStoreName=limit_vel_up  ReadBeforeWriteMsg=warning  WriteAfterWriteMsg=warning  WriteAfterReadMsg=warning  InitialValue=limit_vel_up  ShowAdditionalParam=off  OutDataTypeStr=double
  limit_yaw : DataStoreMemory  DataStoreName=limit_yaw  ReadBeforeWriteMsg=warning  WriteAfterWriteMsg=warning  WriteAfterReadMsg=warning  InitialValue=limit_yaw  VectorParams1D=off  ShowAdditionalParam=off  OutDataTypeStr=double
  mode : DataStoreMemory  DataStoreName=mode  ReadBeforeWriteMsg=warning  WriteAfterWriteMsg=warning  WriteAfterReadMsg=warning  InitialValue=mode  VectorParams1D=off  ShowAdditionalParam=off  OutDataTypeStr=double
  mode_fy : DataStoreMemory  DataStoreName=mode_fy  ReadBeforeWriteMsg=warning  WriteAfterWriteMsg=warning  WriteAfterReadMsg=warning  InitialValue=mode_fy  VectorParams1D=off  ShowAdditionalParam=off  OutDataTypeStr=double
  motors_limit_roll_pitch : DataStoreMemory  DataStoreName=motors_limit_roll_pitch  ReadBeforeWriteMsg=warning  WriteAfterWriteMsg=warning  WriteAfterReadMsg=warning  InitialValue=motors_limit_roll_pitch  VectorParams1D=off  ShowAdditionalParam=off  OutDataTypeStr=double
  motors_limit_throttle_upper : DataStoreMemory  DataStoreName=motors_limit_throttle_upper  ReadBeforeWriteMsg=warning  WriteAfterWriteMsg=warning  WriteAfterReadMsg=warning  InitialValue=motors_limit_throttle_upper  VectorParams1D=off  ShowAdditionalParam=off  OutDataTypeStr=double
  motors_limit_yaw : DataStoreMemory  DataStoreName=motors_limit_yaw  ReadBeforeWriteMsg=warning  WriteAfterWriteMsg=warning  WriteAfterReadMsg=warning  InitialValue=motors_limit_yaw  VectorParams1D=off  ShowAdditionalParam=off  OutDataTypeStr=double
  p_angle_pitch : DataStoreMemory  DataStoreName=p_angle_pitch  ReadBeforeWriteMsg=warning  WriteAfterWriteMsg=warning  WriteAfterReadMsg=warning  InitialValue=p_angle_pitch  VectorParams1D=off  ShowAdditionalParam=off  OutDataTypeStr=double
  p_angle_roll : DataStoreMemory  DataStoreName=p_angle_roll  ReadBeforeWriteMsg=warning  WriteAfterWriteMsg=warning  WriteAfterReadMsg=warning  InitialValue=p_angle_roll  ShowAdditionalParam=off  OutDataTypeStr=double
  p_angle_yaw : DataStoreMemory  DataStoreName=p_angle_yaw  ReadBeforeWriteMsg=warning  WriteAfterWriteMsg=warning  WriteAfterReadMsg=warning  InitialValue=p_angle_yaw  ShowAdditionalParam=off  OutDataTypeStr=double
  pid_accel_z_derivative : DataStoreMemory  DataStoreName=pid_accel_z_derivative  ReadBeforeWriteMsg=warning  WriteAfterWriteMsg=warning  WriteAfterReadMsg=warning  InitialValue=pid_accel_z_derivative  VectorParams1D=off  ShowAdditionalParam=off  OutDataTypeStr=double
  pid_accel_z_input : DataStoreMemory  DataStoreName=pid_accel_z_input  ReadBeforeWriteMsg=warning  WriteAfterWriteMsg=warning  WriteAfterReadMsg=warning  InitialValue=pid_accel_z_input  VectorParams1D=off  ShowAdditionalParam=off  OutDataTypeStr=double
  pid_accel_z_integrator : DataStoreMemory  DataStoreName=pid_accel_z_integrator  ReadBeforeWriteMsg=warning  WriteAfterWriteMsg=warning  WriteAfterReadMsg=warning  InitialValue=pid_accel_z_integrator  VectorParams1D=off  ShowAdditionalParam=off  OutDataTypeStr=double
  pid_accel_z_reset_filter : DataStoreMemory  DataStoreName=pid_accel_z_reset_filter  ReadBeforeWriteMsg=warning  WriteAfterWriteMsg=warning  WriteAfterReadMsg=warning  InitialValue=pid_accel_z_reset_filter  VectorParams1D=off  ShowAdditionalParam=off  OutDataTypeStr=double
  pid_vel_xy_derivative : DataStoreMemory  DataStoreName=pid_vel_xy_derivative  ReadBeforeWriteMsg=warning  WriteAfterWriteMsg=warning  WriteAfterReadMsg=warning  InitialValue=pid_vel_xy_derivative  VectorParams1D=off  ShowAdditionalParam=off  OutDataTypeStr=double
  pid_vel_xy_input : DataStoreMemory  DataStoreName=pid_vel_xy_input  ReadBeforeWriteMsg=warning  WriteAfterWriteMsg=warning  WriteAfterReadMsg=warning  InitialValue=pid_vel_xy_input  VectorParams1D=off  ShowAdditionalParam=off  OutDataTypeStr=double
  pid_vel_xy_integrator : DataStoreMemory  DataStoreName=pid_vel_xy_integrator  ReadBeforeWriteMsg=warning  WriteAfterWriteMsg=warning  WriteAfterReadMsg=warning  InitialValue=pid_vel_xy_integrator  VectorParams1D=off  ShowAdditionalParam=off  OutDataTypeStr=double
  pid_vel_xy_reset_filter : DataStoreMemory  DataStoreName=pid_vel_xy_reset_filter  ReadBeforeWriteMsg=warning  WriteAfterWriteMsg=warning  WriteAfterReadMsg=warning  InitialValue=pid_vel_xy_reset_filter  VectorParams1D=off  ShowAdditionalParam=off  OutDataTypeStr=double
  pitch : DataStoreMemory  DataStoreName=pitch  ReadBeforeWriteMsg=warning  WriteAfterWriteMsg=warning  WriteAfterReadMsg=warning  InitialValue=pitch  VectorParams1D=off  ShowAdditionalParam=off  OutDataTypeStr=double
  pitch_factor : DataStoreMemory  DataStoreName=pitch_factor  ReadBeforeWriteMsg=warning  WriteAfterWriteMsg=warning  WriteAfterReadMsg=warning  InitialValue=pitch_factor  VectorParams1D=off  ShowAdditionalParam=off  OutDataTypeStr=double
  pitch_in : DataStoreMemory  DataStoreName=pitch_in  ReadBeforeWriteMsg=warning  WriteAfterWriteMsg=warning  WriteAfterReadMsg=warning  InitialValue=pitch_in  VectorParams1D=off  ShowAdditionalParam=off  OutDataTypeStr=double
  pitch_target : DataStoreMemory  DataStoreName=pitch_target  ReadBeforeWriteMsg=warning  WriteAfterWriteMsg=warning  WriteAfterReadMsg=warning  InitialValue=pitch_target  VectorParams1D=off  ShowAdditionalParam=off  OutDataTypeStr=double
  pos_error : DataStoreMemory  DataStoreName=pos_error  ReadBeforeWriteMsg=warning  WriteAfterWriteMsg=warning  WriteAfterReadMsg=warning  InitialValue=pos_error  VectorParams1D=off  ShowAdditionalParam=off  OutDataTypeStr=double
  pos_target : DataStoreMemory  DataStoreName=pos_target  ReadBeforeWriteMsg=warning  WriteAfterWriteMsg=warning  WriteAfterReadMsg=warning  InitialValue=pos_target  VectorParams1D=off  ShowAdditionalParam=off  OutDataTypeStr=double
  pwm_max : DataStoreMemory  DataStoreName=pwm_max  ReadBeforeWriteMsg=warning  WriteAfterWriteMsg=warning  WriteAfterReadMsg=warning  InitialValue=pwm_max  VectorParams1D=off  ShowAdditionalParam=off  OutDataTypeStr=double
  pwm_min : DataStoreMemory  DataStoreName=pwm_min  ReadBeforeWriteMsg=warning  WriteAfterWriteMsg=warning  WriteAfterReadMsg=warning  InitialValue=pwm_min  VectorParams1D=off  ShowAdditionalParam=off  OutDataTypeStr=double
  pwm_out : DataStoreMemory  DataStoreName=pwm_out  ReadBeforeWriteMsg=warning  WriteAfterWriteMsg=warning  WriteAfterReadMsg=warning  InitialValue=pwm_out  VectorParams1D=off  ShowAdditionalParam=off  OutDataTypeStr=double
  rate_bf_ff_enabled : DataStoreMemory  DataStoreName=rate_bf_ff_enabled  ReadBeforeWriteMsg=warning  WriteAfterWriteMsg=warning  WriteAfterReadMsg=warning  InitialValue=rate_bf_ff_enabled  ShowAdditionalParam=off  OutDataTypeStr=double
  rate_pitch_pid_derivative : DataStoreMemory  DataStoreName=rate_pitch_pid_derivative  ReadBeforeWriteMsg=warning  WriteAfterWriteMsg=warning  WriteAfterReadMsg=warning  InitialValue=rate_pitch_pid_derivative  VectorParams1D=off  ShowAdditionalParam=off  OutDataTypeStr=double
  rate_pitch_pid_input : DataStoreMemory  DataStoreName=rate_pitch_pid_input  ReadBeforeWriteMsg=warning  WriteAfterWriteMsg=warning  WriteAfterReadMsg=warning  InitialValue=rate_pitch_pid_input  VectorParams1D=off  ShowAdditionalParam=off  OutDataTypeStr=double
  rate_pitch_pid_integrator : DataStoreMemory  DataStoreName=rate_pitch_pid_integrator  ReadBeforeWriteMsg=warning  WriteAfterWriteMsg=warning  WriteAfterReadMsg=warning  InitialValue=rate_pitch_pid_integrator  VectorParams1D=off  ShowAdditionalParam=off  OutDataTypeStr=double
  rate_pitch_pid_reset_filter : DataStoreMemory  DataStoreName=rate_pitch_pid_reset_filter  ReadBeforeWriteMsg=warning  WriteAfterWriteMsg=warning  WriteAfterReadMsg=warning  InitialValue=rate_pitch_pid_reset_filter  VectorParams1D=off  ShowAdditionalParam=off  OutDataTypeStr=double
  rate_roll_pid_derivative : DataStoreMemory  DataStoreName=rate_roll_pid_derivative  ReadBeforeWriteMsg=warning  WriteAfterWriteMsg=warning  WriteAfterReadMsg=warning  InitialValue=rate_roll_pid_derivative  VectorParams1D=off  ShowAdditionalParam=off  OutDataTypeStr=double
  rate_roll_pid_input : DataStoreMemory  DataStoreName=rate_roll_pid_input  ReadBeforeWriteMsg=warning  WriteAfterWriteMsg=warning  WriteAfterReadMsg=warning  InitialValue=rate_roll_pid_input  VectorParams1D=off  ShowAdditionalParam=off  OutDataTypeStr=double
  rate_roll_pid_integrator : DataStoreMemory  DataStoreName=rate_roll_pid_integrator  ReadBeforeWriteMsg=warning  WriteAfterWriteMsg=warning  WriteAfterReadMsg=warning  InitialValue=rate_roll_pid_integrator  VectorParams1D=off  ShowAdditionalParam=off  OutDataTypeStr=double
  rate_roll_pid_reset_filter : DataStoreMemory  DataStoreName=rate_roll_pid_reset_filter  ReadBeforeWriteMsg=warning  WriteAfterWriteMsg=warning  WriteAfterReadMsg=warning  InitialValue=rate_roll_pid_reset_filter  VectorParams1D=off  ShowAdditionalParam=off  OutDataTypeStr=double
  rate_target_ang_vel : DataStoreMemory  DataStoreName=rate_target_ang_vel  ReadBeforeWriteMsg=warning  WriteAfterWriteMsg=warning  WriteAfterReadMsg=warning  InitialValue=rate_target_ang_vel  VectorParams1D=off  ShowAdditionalParam=off  OutDataTypeStr=double
  rate_yaw_pid_derivative : DataStoreMemory  DataStoreName=rate_yaw_pid_derivative  ReadBeforeWriteMsg=warning  WriteAfterWriteMsg=warning  WriteAfterReadMsg=warning  InitialValue=rate_yaw_pid_derivative  VectorParams1D=off  ShowAdditionalParam=off  OutDataTypeStr=double
  rate_yaw_pid_input : DataStoreMemory  DataStoreName=rate_yaw_pid_input  ReadBeforeWriteMsg=warning  WriteAfterWriteMsg=warning  WriteAfterReadMsg=warning  InitialValue=rate_yaw_pid_input  VectorParams1D=off  ShowAdditionalParam=off  OutDataTypeStr=double
  rate_yaw_pid_integrator : DataStoreMemory  DataStoreName=rate_yaw_pid_integrator  ReadBeforeWriteMsg=warning  WriteAfterWriteMsg=warning  WriteAfterReadMsg=warning  InitialValue=rate_roll_pid_integrator  VectorParams1D=off  ShowAdditionalParam=off  OutDataTypeStr=double
  rate_yaw_pid_reset_filter : DataStoreMemory  DataStoreName=rate_yaw_pid_reset_filter  ReadBeforeWriteMsg=warning  WriteAfterWriteMsg=warning  WriteAfterReadMsg=warning  InitialValue=rate_yaw_pid_reset_filter  VectorParams1D=off  ShowAdditionalParam=off  OutDataTypeStr=double
  recalc_leash_xy : DataStoreMemory  DataStoreName=recalc_leash_xy  ReadBeforeWriteMsg=warning  WriteAfterWriteMsg=warning  WriteAfterReadMsg=warning  InitialValue=recalc_leash_xy  VectorParams1D=off  ShowAdditionalParam=off  OutDataTypeStr=double
  recalc_leash_z : DataStoreMemory  DataStoreName=recalc_leash_z  ReadBeforeWriteMsg=warning  WriteAfterWriteMsg=warning  WriteAfterReadMsg=warning  InitialValue=recalc_leash_z  ShowAdditionalParam=off  OutDataTypeStr=double
  reset_accel_to_lean_xy : DataStoreMemory  DataStoreName=reset_accel_to_lean_xy  ReadBeforeWriteMsg=warning  WriteAfterWriteMsg=warning  WriteAfterReadMsg=warning  InitialValue=reset_accel_to_lean_xy  VectorParams1D=off  ShowAdditionalParam=off  OutDataTypeStr=double
  reset_accel_to_throttle : DataStoreMemory  DataStoreName=reset_accel_to_throttle  ReadBeforeWriteMsg=warning  WriteAfterWriteMsg=warning  WriteAfterReadMsg=warning  InitialValue=reset_accel_to_throttle  VectorParams1D=off  ShowAdditionalParam=off  OutDataTypeStr=double
  reset_desired_vel_to_pos : DataStoreMemory  DataStoreName=reset_desired_vel_to_pos  ReadBeforeWriteMsg=warning  WriteAfterWriteMsg=warning  WriteAfterReadMsg=warning  InitialValue=reset_desired_vel_to_pos  VectorParams1D=off  ShowAdditionalParam=off  OutDataTypeStr=double
  reset_rate_to_accel_z : DataStoreMemory  DataStoreName=reset_rate_to_accel_z  ReadBeforeWriteMsg=warning  WriteAfterWriteMsg=warning  WriteAfterReadMsg=warning  InitialValue=reset_rate_to_accel_z  VectorParams1D=off  ShowAdditionalParam=off  OutDataTypeStr=double
  roll : DataStoreMemory  DataStoreName=roll  ReadBeforeWriteMsg=warning  WriteAfterWriteMsg=warning  WriteAfterReadMsg=warning  InitialValue=roll  VectorParams1D=off  ShowAdditionalParam=off  OutDataTypeStr=double
  roll_factor : DataStoreMemory  DataStoreName=roll_factor  ReadBeforeWriteMsg=warning  WriteAfterWriteMsg=warning  WriteAfterReadMsg=warning  InitialValue=roll_factor  VectorParams1D=off  ShowAdditionalParam=off  OutDataTypeStr=double
  roll_in : DataStoreMemory  DataStoreName=roll_in  ReadBeforeWriteMsg=warning  WriteAfterWriteMsg=warning  WriteAfterReadMsg=warning  InitialValue=roll_in  VectorParams1D=off  ShowAdditionalParam=off  OutDataTypeStr=double
  roll_target : DataStoreMemory  DataStoreName=roll_target  ReadBeforeWriteMsg=warning  WriteAfterWriteMsg=warning  WriteAfterReadMsg=warning  InitialValue=roll_target  VectorParams1D=off  ShowAdditionalParam=off  OutDataTypeStr=double
  rot_body_to_ned : DataStoreMemory  DataStoreName=rot_body_to_ned  ReadBeforeWriteMsg=warning  WriteAfterWriteMsg=warning  WriteAfterReadMsg=warning  InitialValue=rot_body_to_ned  VectorParams1D=off  ShowAdditionalParam=off  OutDataTypeStr=double
  slew_yaw : DataStoreMemory  DataStoreName=slew_yaw  ReadBeforeWriteMsg=warning  WriteAfterWriteMsg=warning  WriteAfterReadMsg=warning  InitialValue=slew_yaw  VectorParams1D=off  ShowAdditionalParam=off  OutDataTypeStr=double
  target_yaw_rate : DataStoreMemory  DataStoreName=target_yaw_rate  ReadBeforeWriteMsg=warning  WriteAfterWriteMsg=warning  WriteAfterReadMsg=warning  InitialValue=target_yaw_rate  VectorParams1D=off  ShowAdditionalParam=off  OutDataTypeStr=double
  throttle_avg_max : DataStoreMemory  DataStoreName=throttle_avg_max  ReadBeforeWriteMsg=warning  WriteAfterWriteMsg=warning  WriteAfterReadMsg=warning  InitialValue=throttle_avg_max  VectorParams1D=off  ShowAdditionalParam=off  OutDataTypeStr=double
  throttle_cutoff_frequency : DataStoreMemory  DataStoreName=throttle_cutoff_frequency  ReadBeforeWriteMsg=warning  WriteAfterWriteMsg=warning  WriteAfterReadMsg=warning  InitialValue=throttle_cutoff_frequency  VectorParams1D=off  ShowAdditionalParam=off  OutDataTypeStr=double
  throttle_filter : DataStoreMemory  DataStoreName=throttle_filter  ReadBeforeWriteMsg=warning  WriteAfterWriteMsg=warning  WriteAfterReadMsg=warning  InitialValue=throttle_filter  VectorParams1D=off  ShowAdditionalParam=off  OutDataTypeStr=double
  throttle_hover : DataStoreMemory  DataStoreName=throttle_hover  ReadBeforeWriteMsg=warning  WriteAfterWriteMsg=warning  WriteAfterReadMsg=warning  InitialValue=throttle_hover  VectorParams1D=off  ShowAdditionalParam=off  OutDataTypeStr=double
  throttle_in : DataStoreMemory  DataStoreName=throttle_in  ReadBeforeWriteMsg=warning  WriteAfterWriteMsg=warning  WriteAfterReadMsg=warning  InitialValue=throttle_in  VectorParams1D=off  ShowAdditionalParam=off  OutDataTypeStr=double
  throttle_input : DataStoreMemory  DataStoreName=throttle_input  ReadBeforeWriteMsg=warning  WriteAfterWriteMsg=warning  WriteAfterReadMsg=warning  InitialValue=throttle_input  VectorParams1D=off  ShowAdditionalParam=off  OutDataTypeStr=double
  throttle_lower : DataStoreMemory  DataStoreName=throttle_lower  ReadBeforeWriteMsg=warning  WriteAfterWriteMsg=warning  WriteAfterReadMsg=warning  InitialValue=throttle_lower  VectorParams1D=off  ShowAdditionalParam=off  OutDataTypeStr=double
  throttle_rpy_mix : DataStoreMemory  DataStoreName=throttle_rpy_mix  ReadBeforeWriteMsg=warning  WriteAfterWriteMsg=warning  WriteAfterReadMsg=warning  InitialValue=throttle_rpy_mix  VectorParams1D=off  ShowAdditionalParam=off  OutDataTypeStr=double
  throttle_rpy_mix_desired : DataStoreMemory  DataStoreName=throttle_rpy_mix_desired  ReadBeforeWriteMsg=warning  WriteAfterWriteMsg=warning  WriteAfterReadMsg=warning  InitialValue=throttle_rpy_mix_desired  VectorParams1D=off  ShowAdditionalParam=off  OutDataTypeStr=double
  throttle_thrust_max : DataStoreMemory  DataStoreName=throttle_thrust_max  ReadBeforeWriteMsg=warning  WriteAfterWriteMsg=warning  WriteAfterReadMsg=warning  InitialValue=throttle_thrust_max  VectorParams1D=off  ShowAdditionalParam=off  OutDataTypeStr=double
  throttle_upper : DataStoreMemory  DataStoreName=throttle_upper  ReadBeforeWriteMsg=warning  WriteAfterWriteMsg=warning  WriteAfterReadMsg=warning  InitialValue=throttle_upper  VectorParams1D=off  ShowAdditionalParam=off  OutDataTypeStr=double
  thrust_boost : DataStoreMemory  DataStoreName=thrust_boost  ReadBeforeWriteMsg=warning  WriteAfterWriteMsg=warning  WriteAfterReadMsg=warning  InitialValue=thrust_boost  VectorParams1D=off  ShowAdditionalParam=off  OutDataTypeStr=double
  thrust_boost_ratio : DataStoreMemory  DataStoreName=thrust_boost_ratio  ReadBeforeWriteMsg=warning  WriteAfterWriteMsg=warning  WriteAfterReadMsg=warning  InitialValue=thrust_boost_ratio  VectorParams1D=off  ShowAdditionalParam=off  OutDataTypeStr=double
  thrust_error_angle : DataStoreMemory  DataStoreName=thrust_error_angle  ReadBeforeWriteMsg=warning  WriteAfterWriteMsg=warning  WriteAfterReadMsg=warning  InitialValue=thrust_error_angle  VectorParams1D=off  ShowAdditionalParam=off  OutDataTypeStr=double
  thrust_rpyt_out : DataStoreMemory  DataStoreName=thrust_rpyt_out  ReadBeforeWriteMsg=warning  WriteAfterWriteMsg=warning  WriteAfterReadMsg=warning  InitialValue=thrust_rpyt_out  VectorParams1D=off  ShowAdditionalParam=off  OutDataTypeStr=double
  thrust_slew_time : DataStoreMemory  DataStoreName=thrust_slew_time  ReadBeforeWriteMsg=warning  WriteAfterWriteMsg=warning  WriteAfterReadMsg=warning  InitialValue=thrust_slew_time  VectorParams1D=off  ShowAdditionalParam=off  OutDataTypeStr=double
  use_desvel_ff_z : DataStoreMemory  DataStoreName=use_desvel_ff_z  ReadBeforeWriteMsg=warning  WriteAfterWriteMsg=warning  WriteAfterReadMsg=warning  InitialValue=use_desvel_ff_z  VectorParams1D=off  ShowAdditionalParam=off  OutDataTypeStr=double
  use_sqrt_controller : DataStoreMemory  DataStoreName=use_sqrt_controller  ReadBeforeWriteMsg=warning  WriteAfterWriteMsg=warning  WriteAfterReadMsg=warning  InitialValue=use_sqrt_controller  ShowAdditionalParam=off  OutDataTypeStr=double
  vel_desired : DataStoreMemory  DataStoreName=vel_desired  ReadBeforeWriteMsg=warning  WriteAfterWriteMsg=warning  WriteAfterReadMsg=warning  InitialValue=vel_desired  VectorParams1D=off  ShowAdditionalParam=off  OutDataTypeStr=double
  vel_error : DataStoreMemory  DataStoreName=vel_error  ReadBeforeWriteMsg=warning  WriteAfterWriteMsg=warning  WriteAfterReadMsg=warning  InitialValue=vel_error  VectorParams1D=off  ShowAdditionalParam=off  OutDataTypeStr=double
  vel_error_input : DataStoreMemory  DataStoreName=vel_error_input  ReadBeforeWriteMsg=warning  WriteAfterWriteMsg=warning  WriteAfterReadMsg=warning  InitialValue=vel_error_input  VectorParams1D=off  ShowAdditionalParam=off  OutDataTypeStr=double
  vel_last : DataStoreMemory  DataStoreName=vel_last  ReadBeforeWriteMsg=warning  WriteAfterWriteMsg=warning  WriteAfterReadMsg=warning  InitialValue=vel_last  VectorParams1D=off  ShowAdditionalParam=off  OutDataTypeStr=double
  vel_target : DataStoreMemory  DataStoreName=vel_target  ReadBeforeWriteMsg=warning  WriteAfterWriteMsg=warning  WriteAfterReadMsg=warning  InitialValue=vel_target  VectorParams1D=off  ShowAdditionalParam=off  OutDataTypeStr=double
  xe,ye,ze : Integrator  InitialCondition=[0 0 0]  LimitOutput=on  UpperSaturationLimit=[inf inf 0]  LowerSaturationLimit=[-inf -inf -inf]
  yaw : DataStoreMemory  DataStoreName=yaw  ReadBeforeWriteMsg=warning  WriteAfterWriteMsg=warning  WriteAfterReadMsg=warning  InitialValue=yaw  VectorParams1D=off  ShowAdditionalParam=off  OutDataTypeStr=double
  yaw_factor : DataStoreMemory  DataStoreName=yaw_factor  ReadBeforeWriteMsg=warning  WriteAfterWriteMsg=warning  WriteAfterReadMsg=warning  InitialValue=yaw_factor  VectorParams1D=off  ShowAdditionalParam=off  OutDataTypeStr=double
  yaw_headroom : DataStoreMemory  DataStoreName=yaw_headroom  ReadBeforeWriteMsg=warning  WriteAfterWriteMsg=warning  WriteAfterReadMsg=warning  InitialValue=yaw_headroom  VectorParams1D=off  ShowAdditionalParam=off  OutDataTypeStr=double
  yaw_in : DataStoreMemory  DataStoreName=yaw_in  ReadBeforeWriteMsg=warning  WriteAfterWriteMsg=warning  WriteAfterReadMsg=warning  InitialValue=yaw_in  VectorParams1D=off  ShowAdditionalParam=off  OutDataTypeStr=double
  z_accel_meas : DataStoreMemory  DataStoreName=z_accel_meas  ReadBeforeWriteMsg=warning  WriteAfterWriteMsg=warning  WriteAfterReadMsg=warning  InitialValue=z_accel_meas  VectorParams1D=off  ShowAdditionalParam=off  OutDataTypeStr=double
  wires:
  6DOF (Euler Angles)/4 -> Transpose/1, Inertial to Body/1
  Data Store Read/1 -> Scope3/1, Display7/1, MATLAB Function/1(pwm_out)
  Inertial to Body/1 -> Scope62/1, Gain8/1, Gravity in Earth Axes/1
  MATLAB Function/1(F) -> Scope58/1, 6DOF (Euler Angles)/1
  MATLAB Function/2(M) -> 6DOF (Euler Angles)/2
  6DOF (Euler Angles)/1 -> xe,ye,ze/1, curr_vel_limt/1(Ve)
  xe,ye,ze/1 -> curr_vel_limt/2(Xe), Demux11/1, Gain7/1
  6DOF (Euler Angles)/5 -> Scope59/1
  6DOF (Euler Angles)/8 -> Add3/1
  6DOF (Euler Angles)/3 -> Demux/1
  Demux/1 -> Data Store Write1/1
  Demux/3 -> Data Store Write2/1
  Data Store Read1/1 -> Gain/1
  Data Store Read3/1 -> Scope24/1, Display11/1
  Data Store Read4/1 -> Display12/1
  Demux/2 -> Data Store Write3/1
  Data Store Read5/1 -> Display5/1
  Gain/1 -> Scope/1, Display10/1
  Data Store Read6/1 -> Display13/1
  Data Store Read7/1 -> Gain1/1
  Gain1/1 -> Display14/1
  Data Store Read9/1 -> Scope1/1
  Data Store Read10/1 -> Scope2/1, Gain2/1
  6DOF (Euler Angles)/6 -> Scope10/1, Demux1/1, Display17/1
  Demux1/2 -> Data Store Write5/1, Scope12/1
  Gain2/1 -> Display15/1
  Data Store Read8/1 -> Scope22/1, Display4/1
  Data Store Read11/1 -> Scope25/1, Display16/1
  Data Store Read12/1 -> Demux2/1, Gain3/1
  Gain3/1 -> Display18/1
  Demux2/2 -> Scope2/2
  Data Store Read13/1 -> Scope4/1
  Data Store Read14/1 -> Scope5/1
  Data Store Read15/1 -> Scope6/1
  Data Store Read17/1 -> Scope7/1
  Data Store Read16/1 -> Scope60/3, Scope8/1
  Demux1/3 -> Scope11/1, Data Store Write6/1
  Demux1/1 -> Data Store Write4/1, Scope13/1
  Data Store Read18/1 -> Scope15/1
  Data Store Read21/1 -> Scope16/1
  Data Store Read20/1 -> Scope17/1
  Data Store Read22/1 -> MATLAB Function1/1(q)
  Demux3/2 -> Scope18/1
  MATLAB Function1/1(euler_angle) -> Demux3/1
  Demux4/2 -> Scope18/2, Scope19/1
  Data Store Read23/1 -> Demux4/1
  Data Store Read24/1 -> Scope57/2, Add/2
  Add/1 -> Product/1, Scope18/3, Scope20/1
  Data Store Read25/1 -> Demux5/1
  Data Store Read26/1 -> Scope21/1, Demux6/1
  Demux6/2 -> Scope20/3
  Constant/1 -> Product/2
  Product/1 -> Scope20/2
  Data Store Read2/1 -> Scope23/1, Display2/1
  Demux2/1 -> Scope22/2
  Demux2/3 -> Scope25/2
  Product1/1 -> Scope28/2
  Constant1/1 -> Product1/2
  Demux10/3 -> Scope28/3
  Data Store Read31/1 -> Demux10/1, Scope29/1
  Demux9/3 -> Add1/1
  Data Store Read30/1 -> Demux9/1
  Add1/1 -> Scope28/1, Scope26/3, Product1/1
  Data Store Read29/1 -> Add1/2
  Data Store Read28/1 -> Demux8/1
  Demux8/3 -> Scope26/2, Scope27/1
  MATLAB Function2/1(euler_angle) -> Demux7/1
  Demux7/3 -> Scope26/1
  Data Store Read27/1 -> MATLAB Function2/1(q)
  Demux11/3 -> Gain4/1
  Gain4/1 -> Scope30/1, Data Store Write7/1
  Data Store Read32/1 -> Scope31/1
  Data Store Read33/1 -> Scope32/1
  Demux23/3 -> Gain6/1
  Data Store Read34/1 -> Demux12/1
  Demux12/2 -> Scope33/2, Scope65/1
  Demux12/1 -> Scope66/1, Scope33/1
  Demux12/3 -> Scope38/1, Scope33/3
  Data Store Read36/1 -> Demux13/1
  Demux13/3 -> Scope38/3, Scope35/1
  Gain5/1 -> Data Store Write9/1
  Data Store Read40/1 -> Scope41/1
  Demux21/3 -> Scope53/3, Scope42/1
  Data Store Read43/1 -> Add2/2, Scope51/2, Scope44/1
  Data Store Read44/1 -> Demux15/1
  Data Store Read45/1 -> Demux14/1
  Demux14/3 -> Scope52/2, Scope51/3, Scope46/1
  Demux15/3 -> Scope45/1
  Data Store Read42/1 -> Demux16/1
  Demux16/3 -> Scope51/1, Add2/1, Scope43/1
  Transpose/1 -> Inertial to NED/1
  Add3/1 -> Demux17/1, Inertial to NED/2
  Add2/1 -> Scope52/1
  Data Store Read46/1 -> Scope54/1
  Gain7/1 -> Display1/1, Demux18/1, Data Store Write10/1, Scope55/1
  Demux18/1 -> Scope56/1
  Demux18/2 -> Scope56/2
  Demux5/2 -> Scope57/1, Add/1
  Demux18/3 -> Scope56/3
  Data Store Read48/1 -> Cos/1
  Cos/1 -> Divide/2
  Constant2/1 -> Divide/1
  Divide/1 -> Scope60/1
  Data Store Read19/1 -> Scope60/2, Scope9/1
  gn/1 -> Scope61/1, Inertial to Body/2
  Data Store Read49/1 -> Scope64/1
  Constant3/1 -> Data Store Write/1
  Gain8/1 -> Add3/2
  Demux17/1 -> Scope48/1, Data Store Write12/1
  Demux17/2 -> Scope49/1, Data Store Write11/1
  Demux17/3 -> Scope50/1, Data Store Write8/1
  Gravity in Earth Axes/1 -> MATLAB Function/2(gn)
  curr_vel_limt/1(Vo) -> Scope39/1, Gain5/1
  Data Store Read37/1 -> Demux19/1
  Demux19/3 -> Scope53/1, Scope36/1
  Data Store Read41/1 -> Demux21/1
  Data Store Read38/1 -> Demux22/1
  Demux22/3 -> Scope53/2, Scope37/1
  Data Store Read39/1 -> Demux20/1
  Demux20/3 -> Scope40/1
  Data Store Read50/1 -> Demux23/1
  Gain6/1 -> Scope38/2, Scope34/1
  Demux23/2 -> Scope65/2
  Demux23/1 -> Scope66/2
  Demux19/1 -> Scope67/1
  Demux22/1 -> Scope67/2
  Demux16/1 -> Scope68/1
  Data Store Read35/1 -> Demux24/1
  Demux24/1 -> Scope14/1
  Demux25/1 -> Scope14/2
  Inertial to NED/1 -> Gain9/1
  Gain9/1 -> Demux25/1
  Demux24/2 -> Scope47/1
  Demux25/2 -> Scope47/2
  Demux24/3 -> Scope63/1
  Demux25/3 -> Scope63/2
